simulink model "modules"  (R2017a)
settings: Solver=ode4  StartTime=0.0  StopTime=time_stop  FixedStep=time_step  RelTol=1e-3
values from neighbouring files (symbols this model uses):
  psi = state(3)    [PSVobstacleShip_class.m]    (also in PSVvessel_class.m = obj.eta(3); PsiReferenceModel_class.m = obj.desired_psi_vector; SBMPC_PSVvessel_class.m = obj.eta(3))
undefined symbols (not defined in the file or in its folder): beta, Delta_guidance, Delta_matrix, eta_initial, initial_desired_psi_vector, initial_desired_u_vector, initial_next_waypoint_indexes, initial_obstacle_ship_states, initial_obstacle_ship_states_dot, initial_reference_psi_vector, initial_reference_u_vector, initial_SBMPC_desired_psi_vector, initial_SBMPC_desired_u_vector, initial_SBMPC_next_waypoint_indexes, initial_SBMPC_obstacle_ship_states, initial_SBMPC_obstacle_ship_states_dot, initial_SBMPC_reference_psi_vector, initial_SBMPC_reference_u_vector, initial_SBMPC_x_d_psi_matrix, initial_SBMPC_x_d_u_matrix, initial_state, initial_x_d_psi_matrix, initial_x_d_u_matrix, K_sway, K_yaw, Kp_feedback_linearization, kp_heading, Nmax, nu_initial, num_obs_ship_waypoints, num_prediction_time_steps, number_of_control_behaviors, number_of_obstacle_ships, number_of_SBMPC_obstacle_ships, obs_speed_between_waypoints, obstacle_waypoint_matrix, Omega_matrix, own_ship_reference_psi_init, own_ship_reference_speed, Psi_init, radius_of_acceptance, SBMPC_obs_speed_between_waypoints, SBMPC_obstacle_waypoint_matrix, seconds_between_prediction, state_vector_init, T, T_k_surge, T_k_sway, T_k_yaw, T_s, T_waypoints, time_step, tsamp, U, U_init, V_init, waypoints_obstacle_ships, waypoints_own_ship, Xmax, Ymax
(part 2 of 5)

== system modules/obstacle ships/guidance  ==
  state matrix : Inport
  "waypoints matrix " : Inport  Port=2
  MATLAB Function1 : MATLAB Function  TreatAsAtomicUnit=on
  Scope : Scope
  Scope1 : Scope
  Scope2 : Scope
  obstacle waypoint guidance : MATLAB Function  TreatAsAtomicUnit=on
  "reference psi " : Outport
  reference u vector : Outport  Port=2
  "next_waypoints_indexes " : Outport  Port=3
  wires:
  "waypoints matrix "/1 -> obstacle waypoint guidance/1(obstacle_waypoints)
  state matrix/1 -> obstacle waypoint guidance/2(state_matrix)
  obstacle waypoint guidance/1(reference_psi_vector) -> "reference psi "/1, Scope/1
  MATLAB Function1/1(u_vector) -> Scope2/1, reference u vector/1
  obstacle waypoint guidance/2(next_waypoints_indexes) -> MATLAB Function1/1(next_waypoints_indexes), Scope1/1, "next_waypoints_indexes "/1

== system modules/obstacle ships/reference model for psi ==
  note: row vector
  note: row vector
  reference psi vector : Inport
  Scope3 : Scope  NumInputPorts=2
  To Workspace : ToWorkspace  VariableName=obstacle_ships_reference_psi_vector  SampleTime=tsamp
      settings: Save2DSignal=2-D array (concatenate along first dimension)
  To Workspace1 : ToWorkspace  VariableName=obstacle_ships_desired_psi_vector  SampleTime=tsamp
      settings: Save2DSignal=2-D array (concatenate along first dimension)
  "psi reference model " : MATLAB Function  TreatAsAtomicUnit=on
  "desired psi vector " : Outport
  wires:
  "psi reference model "/1(desired_psi_vector) -> Scope3/1, To Workspace1/1, "desired psi vector "/1
  reference psi vector/1 -> Scope3/2, To Workspace/1, "psi reference model "/1(reference_psi_vector)

== system modules/obstacle ships/reference model for u ==
  note: row vector
  note: row vector
  "reference u vector " : Inport
  MATLAB Function1 : MATLAB Function  TreatAsAtomicUnit=on
  To Workspace : ToWorkspace  VariableName=obstacle_ships_reference_u_vector  SampleTime=tsamp
      settings: Save2DSignal=2-D array (concatenate along first dimension)
  To Workspace1 : ToWorkspace  VariableName=obstacle_ships_desired_u_vector  SampleTime=tsamp
      settings: Save2DSignal=2-D array (concatenate along first dimension)
  desired_u_vector : Outport
  wires:
  "reference u vector "/1 -> To Workspace/1, MATLAB Function1/1(reference_u_vetor)
  MATLAB Function1/1(desired_u_vector) -> To Workspace1/1, desired_u_vector/1

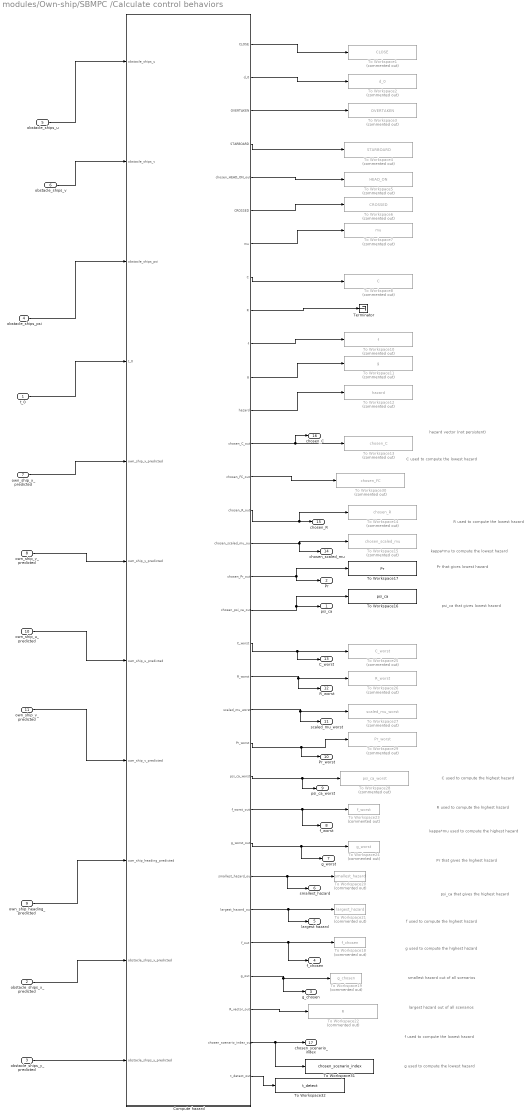
== system modules/Own-ship/SBMPC /Calculate control behaviors ==
  note: hazard vector (not persistent)
  note: C used to compute the lowest hazard
  note: R used to compute the lowest hazard
  note: kappa*mu to compute the lowest hazard
  note: Pr that gives lowest hazard
  note: psi_ca that gives lowest hazard
  note: C used to compute the highest hazard
  note: R used to compute the highest hazard
  note: kappa*mu used to compute the highest hazard
  note: Pr that gives the highest hazard
  note: psi_ca that gives the highest hazard
  note: f used to compute the highest hazard
  note: g used to compute the highest hazard
  note: smallest hazard out of all scenarios
  note: largest hazard out of all scenarios
  note: f used to compute the lowest hazard
  note: g used to compute the lowest hazard
  t_0 : Inport
  obstacle_ships_x_predicted : Inport  Port=2  SampleTime=time_step
      settings: VarSizeSig=Yes
  "obstacle_ships_y_predicted " : Inport  Port=3  SampleTime=time_step
      settings: VarSizeSig=Yes
  obstacle_ships_psi : Inport  Port=4
  obstacle_ships_u : Inport  Port=5
  obstacle_ships_v : Inport  Port=6
  own_ship_x_predicted : Inport  Port=7  SampleTime=time_step
      settings: VarSizeSig=Yes
  own_ship_y_predicted : Inport  Port=8  SampleTime=time_step
      settings: VarSizeSig=Yes
  "own_ship_heading_predicted " : Inport  Port=9  SampleTime=time_step
      settings: VarSizeSig=Yes
  own_ship_u_predicted : Inport  Port=10  SampleTime=time_step
      settings: VarSizeSig=Yes
  "own_ship_v_predicted " : Inport  Port=11  SampleTime=time_step
      settings: VarSizeSig=Yes
  Compute hazard : MATLAB Function  TreatAsAtomicUnit=on
  Terminator : Terminator
  To Workspace1 : ToWorkspace  Commented=on  VariableName=CLOSE  SaveFormat=Structure With Time  SampleTime=tsamp
  To Workspace10 : ToWorkspace  Commented=on  VariableName=f  SaveFormat=Structure With Time  SampleTime=tsamp
      settings: Save2DSignal=2-D array (concatenate along first dimension)
  To Workspace11 : ToWorkspace  Commented=on  VariableName=g  SaveFormat=Structure With Time  SampleTime=tsamp
  To Workspace12 : ToWorkspace  Commented=on  VariableName=hazard  SaveFormat=Structure With Time  SampleTime=tsamp
      settings: Save2DSignal=2-D array (concatenate along first dimension)
  To Workspace13 : ToWorkspace  Commented=on  VariableName=chosen_C  SampleTime=tsamp
      settings: Save2DSignal=2-D array (concatenate along first dimension)
  To Workspace14 : ToWorkspace  Commented=on  VariableName=chosen_R  SampleTime=tsamp
      settings: Save2DSignal=2-D array (concatenate along first dimension)
  To Workspace15 : ToWorkspace  Commented=on  VariableName=chosen_scaled_mu  SampleTime=tsamp
      settings: Save2DSignal=2-D array (concatenate along first dimension)
  To Workspace16 : ToWorkspace  VariableName=psi_ca  SampleTime=tsamp
      settings: Save2DSignal=2-D array (concatenate along first dimension)
  To Workspace17 : ToWorkspace  VariableName=Pr  SampleTime=tsamp
      settings: Save2DSignal=2-D array (concatenate along first dimension)
  To Workspace18 : ToWorkspace  Commented=on  VariableName=f_chosen  SampleTime=tsamp
      settings: Save2DSignal=2-D array (concatenate along first dimension)
  To Workspace19 : ToWorkspace  Commented=on  VariableName=g_chosen  SampleTime=tsamp
      settings: Save2DSignal=2-D array (concatenate along first dimension)
  To Workspace2 : ToWorkspace  Commented=on  VariableName=d_0  SaveFormat=Structure With Time  SampleTime=tsamp
  To Workspace20 : ToWorkspace  Commented=on  VariableName=smallest_hazard  SampleTime=tsamp
      settings: Save2DSignal=2-D array (concatenate along first dimension)
  To Workspace21 : ToWorkspace  Commented=on  VariableName=largest_hazard  SampleTime=tsamp
      settings: Save2DSignal=2-D array (concatenate along first dimension)
  To Workspace22 : ToWorkspace  Commented=on  VariableName=R  SaveFormat=Structure With Time  SampleTime=tsamp
  To Workspace23 : ToWorkspace  Commented=on  VariableName=f_worst  SampleTime=tsamp
      settings: Save2DSignal=2-D array (concatenate along first dimension)
  To Workspace24 : ToWorkspace  Commented=on  VariableName=g_worst  SampleTime=tsamp
      settings: Save2DSignal=2-D array (concatenate along first dimension)
  To Workspace25 : ToWorkspace  Commented=on  VariableName=C_worst  SampleTime=tsamp
      settings: Save2DSignal=2-D array (concatenate along first dimension)
  To Workspace26 : ToWorkspace  Commented=on  VariableName=R_worst  SampleTime=tsamp
      settings: Save2DSignal=2-D array (concatenate along first dimension)
  To Workspace27 : ToWorkspace  Commented=on  VariableName=scaled_mu_worst  SampleTime=tsamp
      settings: Save2DSignal=2-D array (concatenate along first dimension)
  To Workspace28 : ToWorkspace  Commented=on  VariableName=psi_ca_worst  SampleTime=tsamp
      settings: Save2DSignal=2-D array (concatenate along first dimension)
  To Workspace29 : ToWorkspace  Commented=on  VariableName=Pr_worst  SampleTime=tsamp
      settings: Save2DSignal=2-D array (concatenate along first dimension)
  To Workspace3 : ToWorkspace  Commented=on  VariableName=OVERTAKEN  SaveFormat=Structure With Time  SampleTime=tsamp
  To Workspace30 : ToWorkspace  Commented=on  VariableName=chosen_FC  SampleTime=tsamp
      settings: Save2DSignal=2-D array (concatenate along first dimension)
  To Workspace31 : ToWorkspace  VariableName=chosen_scenario_index  SampleTime=tsamp
      settings: Save2DSignal=2-D array (concatenate along first dimension)
  To Workspace32 : ToWorkspace  VariableName=t_detect  SaveFormat=Structure With Time  SampleTime=tsamp
      settings: Save2DSignal=2-D array (concatenate along first dimension)
  To Workspace4 : ToWorkspace  Commented=on  VariableName=STARBOARD  SaveFormat=Structure With Time  SampleTime=tsamp
  To Workspace5 : ToWorkspace  Commented=on  VariableName=HEAD_ON  SaveFormat=Structure With Time  SampleTime=tsamp
      settings: Save2DSignal=2-D array (concatenate along first dimension)
  To Workspace6 : ToWorkspace  Commented=on  VariableName=CROSSED  SaveFormat=Structure With Time  SampleTime=tsamp
  To Workspace7 : ToWorkspace  Commented=on  VariableName=mu  SaveFormat=Structure With Time  SampleTime=tsamp
  To Workspace8 : ToWorkspace  Commented=on  VariableName=C  SampleTime=tsamp
  psi_ca : Outport  SampleTime=time_step
  Pr : Outport  Port=2  SampleTime=time_step
  "g_chosen " : Outport  Port=3  SampleTime=time_step
  f_chosen : Outport  Port=4  SampleTime=time_step
  largest hazard : Outport  Port=5  SampleTime=time_step
  smallest_hazard : Outport  Port=6  SampleTime=time_step
  "g_worst " : Outport  Port=7  SampleTime=time_step
  f_worst : Outport  Port=8  SampleTime=time_step
  psi_ca_worst : Outport  Port=9  SampleTime=time_step
  Pr_worst : Outport  Port=10  SampleTime=time_step
  scaled_mu_worst : Outport  Port=11  SampleTime=time_step
  R_worst : Outport  Port=12  SampleTime=time_step
  C_worst : Outport  Port=13  SampleTime=time_step
  chosen_scaled_mu : Outport  Port=14  SampleTime=time_step
  chosen_R : Outport  Port=15  SampleTime=time_step
  chosen_C : Outport  Port=16  SampleTime=time_step
  "chosen_scenario_index " : Outport  Port=17  SampleTime=time_step
  wires:
  own_ship_x_predicted/1 -> Compute hazard/5(own_ship_x_predicted)
  own_ship_y_predicted/1 -> Compute hazard/6(own_ship_y_predicted)
  obstacle_ships_x_predicted/1 -> Compute hazard/10(obstacle_ships_x_predicted)
  "obstacle_ships_y_predicted "/1 -> Compute hazard/11(obstacle_ships_y_predicted)
  t_0/1 -> Compute hazard/4(t_0)
  Compute hazard/1(CLOSE) -> To Workspace1/1
  Compute hazard/2(d_0) -> To Workspace2/1
  obstacle_ships_v/1 -> Compute hazard/2(obstacle_ships_v)
  obstacle_ships_u/1 -> Compute hazard/1(obstacle_ships_u)
  own_ship_u_predicted/1 -> Compute hazard/7(own_ship_u_predicted)
  "own_ship_v_predicted "/1 -> Compute hazard/8(own_ship_v_predicted)
  "own_ship_heading_predicted "/1 -> Compute hazard/9(own_ship_heading_predicted)
  obstacle_ships_psi/1 -> Compute hazard/3(obstacle_ships_psi)
  Compute hazard/3(OVERTAKEN) -> To Workspace3/1
  Compute hazard/4(STARBOARD) -> To Workspace4/1
  Compute hazard/5(chosen_HEAD_ON_out) -> To Workspace5/1
  Compute hazard/6(CROSSED) -> To Workspace6/1
  Compute hazard/7(mu) -> To Workspace7/1
  Compute hazard/12(hazard) -> To Workspace12/1
  Compute hazard/8(C) -> To Workspace8/1
  Compute hazard/10(f) -> To Workspace10/1
  Compute hazard/11(g) -> To Workspace11/1
  Compute hazard/13(chosen_C_out) -> chosen_C/1, To Workspace13/1
  Compute hazard/15(chosen_R_out) -> To Workspace14/1, chosen_R/1
  Compute hazard/16(chosen_scaled_mu_out) -> To Workspace15/1, chosen_scaled_mu/1
  Compute hazard/18(chosen_psi_ca_out) -> To Workspace16/1, psi_ca/1
  Compute hazard/19(C_worst) -> C_worst/1, To Workspace25/1
  Compute hazard/20(R_worst) -> R_worst/1, To Workspace26/1
  Compute hazard/21(scaled_mu_worst) -> scaled_mu_worst/1, To Workspace27/1
  Compute hazard/22(Pr_worst) -> Pr_worst/1, To Workspace29/1
  Compute hazard/23(psi_ca_worst) -> psi_ca_worst/1, To Workspace28/1
  Compute hazard/25(g_worst_out) -> "g_worst "/1, To Workspace24/1
  Compute hazard/24(f_worst_out) -> f_worst/1, To Workspace23/1
  Compute hazard/17(chosen_Pr_out) -> To Workspace17/1, Pr/1
  Compute hazard/28(f_out) -> f_chosen/1, To Workspace18/1
  Compute hazard/29(g_out) -> "g_chosen "/1, To Workspace19/1
  Compute hazard/26(smallest_hazard_out) -> smallest_hazard/1, To Workspace20/1
  Compute hazard/27(largest_hazard_out) -> largest hazard/1, To Workspace21/1
  Compute hazard/30(R_vector_out) -> To Workspace22/1
  Compute hazard/9(R) -> Terminator/1
  Compute hazard/14(chosen_FC_out) -> To Workspace30/1
  Compute hazard/31(chosen_scenario_index_out) -> To Workspace31/1, "chosen_scenario_index "/1
  Compute hazard/32(t_detect_out) -> To Workspace32/1

== system modules/Own-ship/SBMPC /Own-ship trajectory prediction ==
  note: each row = time step in prediction horizion
      | each column = a different control scenario
  note: each row = time step in prediction horizion
      | each column = a different control scenario
  note: each row = time step in prediction horizion
      | each column = a different control scenario
  note: each row = time step in prediction horizion
      | each column = a different control scenario
  note: each row = time step in prediction horizion
      | each column = a different control scenario
  t_0 : Inport
  waypoints_matrix : Inport  Port=2
  "eta_initial " : Inport  Port=3
  nu_initial : Inport  Port=4
  next_waypoint_index : Inport  Port=5
  Own ship trajectory prediction : MATLAB Function  TreatAsAtomicUnit=on
  To Workspace1 : ToWorkspace  Commented=on  VariableName=own_ship_x_predicted  SaveFormat=Structure With Time  SampleTime=tsamp
  To Workspace3 : ToWorkspace  Commented=on  VariableName=own_ship_y_predicted  SaveFormat=Structure With Time  SampleTime=tsamp
  To Workspace4 : ToWorkspace  Commented=on  VariableName=own_ship_heading_predicted  SaveFormat=Structure With Time  SampleTime=tsamp
  To Workspace5 : ToWorkspace  Commented=on  VariableName=own_ship_u_predicted  SaveFormat=Structure With Time  SampleTime=tsamp
  To Workspace6 : ToWorkspace  Commented=on  VariableName=own_ship_v_predicted  SaveFormat=Structure With Time  SampleTime=tsamp
  own_ship_x_predicted : Outport  SampleTime=time_step
  own_ship_y_predicted : Outport  Port=2  SampleTime=time_step
  own_ship_heading_predicted : Outport  Port=3  SampleTime=time_step
  own_ship_u_predicted : Outport  Port=4  SampleTime=time_step
  "own_ship_v_predicted " : Outport  Port=5  SampleTime=time_step
  wires:
  waypoints_matrix/1 -> Own ship trajectory prediction/4(waypoints_matrix)
  nu_initial/1 -> Own ship trajectory prediction/3(nu_initial)
  "eta_initial "/1 -> Own ship trajectory prediction/2(eta_initial)
  next_waypoint_index/1 -> Own ship trajectory prediction/5(next_waypoint_index)
  t_0/1 -> Own ship trajectory prediction/1(t_0)
  Own ship trajectory prediction/1(own_ship_x_predicted) -> own_ship_x_predicted/1, To Workspace1/1
  Own ship trajectory prediction/2(own_ship_y_predicted) -> own_ship_y_predicted/1, To Workspace3/1
  Own ship trajectory prediction/3(own_ship_heading_predicted) -> To Workspace4/1, own_ship_heading_predicted/1
  Own ship trajectory prediction/4(own_ship_u_predicted) -> own_ship_u_predicted/1, To Workspace5/1
  Own ship trajectory prediction/5(own_ship_v_predicted) -> "own_ship_v_predicted "/1, To Workspace6/1

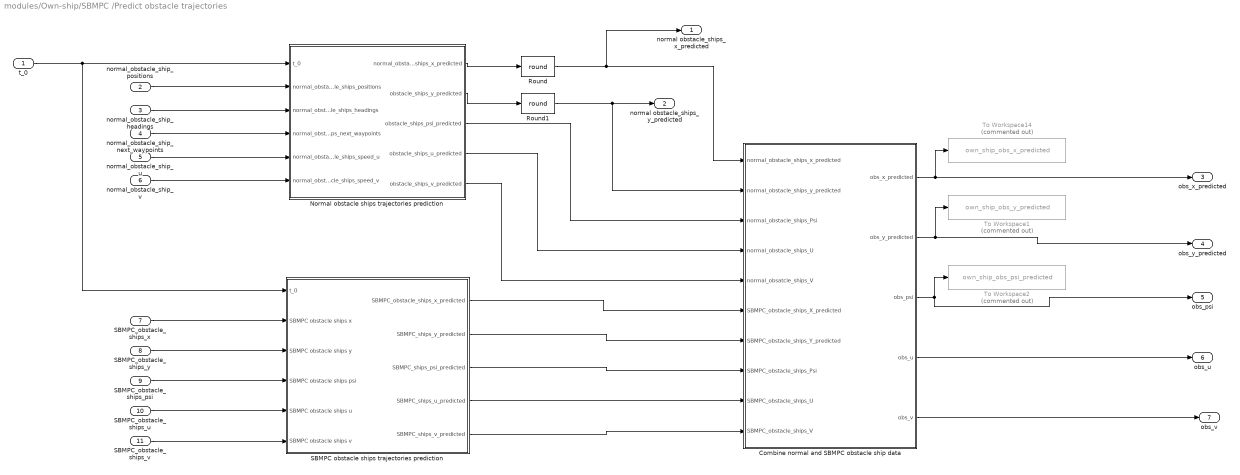
== system modules/Own-ship/SBMPC /Predict obstacle trajectories ==
  t_0 : Inport
  normal_obstacle_ship_positions : Inport  Port=2
  normal_obstacle_ship_headings : Inport  Port=3
  normal_obstacle_ship_next_waypoints : Inport  Port=4
  normal_obstacle_ship_u : Inport  Port=5
  normal_obstacle_ship_v : Inport  Port=6
  SBMPC_obstacle_ships_x : Inport  Port=7
  SBMPC_obstacle_ships_y : Inport  Port=8
  SBMPC_obstacle_ships_psi : Inport  Port=9
  SBMPC_obstacle_ships_u : Inport  Port=10
  SBMPC_obstacle_ships_v : Inport  Port=11
  "Combine normal and SBMPC obstacle ship data " : MATLAB Function  TreatAsAtomicUnit=on
  Normal obstacle ships trajectories prediction : Subsystem
  Round : Rounding  Operator=round
  Round1 : Rounding  Operator=round
  SBMPC obstacle ships trajectories prediction : Subsystem
  To Workspace1 : ToWorkspace  Commented=on  VariableName=own_ship_obs_y_predicted  SaveFormat=Structure With Time  SampleTime=tsamp
      settings: Save2DSignal=2-D array (concatenate along first dimension)
  To Workspace14 : ToWorkspace  Commented=on  VariableName=own_ship_obs_x_predicted  SaveFormat=Structure With Time  SampleTime=tsamp
      settings: Save2DSignal=2-D array (concatenate along first dimension)
  To Workspace2 : ToWorkspace  Commented=on  VariableName=own_ship_obs_psi_predicted  SaveFormat=Structure With Time  SampleTime=tsamp
      settings: Save2DSignal=2-D array (concatenate along first dimension)
  normal obstacle_ships_x_predicted : Outport  SampleTime=time_step
  "normal obstacle_ships_y_predicted " : Outport  Port=2  SampleTime=time_step
  obs_x_predicted : Outport  Port=3
  obs_y_predicted : Outport  Port=4
  obs_psi : Outport  Port=5
  obs_u : Outport  Port=6
  obs_v : Outport  Port=7
  wires:
  Normal obstacle ships trajectories prediction/1(normal_obstacle_ships_x_predicted) -> Round/1
  normal_obstacle_ship_u/1 -> Normal obstacle ships trajectories prediction/5(normal_obstacle_ships_speed_u)
  normal_obstacle_ship_headings/1 -> Normal obstacle ships trajectories prediction/3(normal_obstacle_ships_headings)
  normal_obstacle_ship_positions/1 -> Normal obstacle ships trajectories prediction/2(normal_obstacle_ships_positions)
  Normal obstacle ships trajectories prediction/2(obstacle_ships_y_predicted) -> Round1/1
  normal_obstacle_ship_v/1 -> Normal obstacle ships trajectories prediction/6(normal_obstacle_ships_speed_v)
  "Combine normal and SBMPC obstacle ship data "/5(obs_v) -> obs_v/1
  Normal obstacle ships trajectories prediction/5(obstacle_ships_v_predicted) -> "Combine normal and SBMPC obstacle ship data "/5(normal_obsatcle_ships_V)
  Normal obstacle ships trajectories prediction/4(obstacle_ships_u_predicted) -> "Combine normal and SBMPC obstacle ship data "/4(normal_obstacle_ships_U)
  "Combine normal and SBMPC obstacle ship data "/2(obs_y_predicted) -> obs_y_predicted/1, To Workspace1/1
  "Combine normal and SBMPC obstacle ship data "/1(obs_x_predicted) -> obs_x_predicted/1, To Workspace14/1
  "Combine normal and SBMPC obstacle ship data "/3(obs_psi) -> obs_psi/1, To Workspace2/1
  normal_obstacle_ship_next_waypoints/1 -> Normal obstacle ships trajectories prediction/4(normal_obstacle_ships_next_waypoints)
  Normal obstacle ships trajectories prediction/3(obstacle_ships_psi_predicted) -> "Combine normal and SBMPC obstacle ship data "/3(normal_obstacle_ships_Psi)
  "Combine normal and SBMPC obstacle ship data "/4(obs_u) -> obs_u/1
  SBMPC_obstacle_ships_psi/1 -> SBMPC obstacle ships trajectories prediction/4(SBMPC obstacle ships psi)
  SBMPC_obstacle_ships_u/1 -> SBMPC obstacle ships trajectories prediction/5(SBMPC obstacle ships u)
  SBMPC_obstacle_ships_y/1 -> SBMPC obstacle ships trajectories prediction/3("SBMPC obstacle ships y ")
  SBMPC_obstacle_ships_v/1 -> SBMPC obstacle ships trajectories prediction/6(SBMPC obstacle ships v)
  SBMPC obstacle ships trajectories prediction/3(SBMPC_ships_psi_predicted) -> "Combine normal and SBMPC obstacle ship data "/8(SBMPC_obstacle_ships_Psi)
  SBMPC obstacle ships trajectories prediction/5(SBMPC_ships_v_predicted) -> "Combine normal and SBMPC obstacle ship data "/10(SBMPC_obstacle_ships_V)
  SBMPC obstacle ships trajectories prediction/4(SBMPC_ships_u_predicted) -> "Combine normal and SBMPC obstacle ship data "/9(SBMPC_obstacle_ships_U)
  SBMPC obstacle ships trajectories prediction/2(SBMPC_ships_y_predicted) -> "Combine normal and SBMPC obstacle ship data "/7(SBMPC_obstacle_ships_Y_predicted)
  SBMPC obstacle ships trajectories prediction/1(SBMPC_obstacle_ships_x_predicted) -> "Combine normal and SBMPC obstacle ship data "/6(SBMPC_obstacle_ships_X_predicted)
  SBMPC_obstacle_ships_x/1 -> SBMPC obstacle ships trajectories prediction/2("SBMPC obstacle ships x ")
  t_0/1 -> SBMPC obstacle ships trajectories prediction/1(t_0), Normal obstacle ships trajectories prediction/1(t_0)
  Round/1 -> normal obstacle_ships_x_predicted/1, "Combine normal and SBMPC obstacle ship data "/1(normal_obstacle_ships_x_predicted)
  Round1/1 -> "normal obstacle_ships_y_predicted "/1, "Combine normal and SBMPC obstacle ship data "/2(normal_obstacle_ships_y_predicted)

== system modules/Own-ship/vessel1/Vessel model ==
  desired_nu : Inport
  desired_psi : Inport  Port=2
  Pr : Inport  Port=3
  psi_ca : Inport  Port=4
  Demux : Demux  Outputs=6
  MATLAB Function : MATLAB Function  TreatAsAtomicUnit=on
  Mux : Mux  Inputs=3
  Terminator : Terminator
  To Workspace : ToWorkspace  Commented=on  VariableName=tau  SampleTime=tsamp
      settings: Save2DSignal=2-D array (concatenate along first dimension)
  state : Outport
  x : Outport  Port=2
  y : Outport  Port=3
  psi : Outport  Port=4
  u : Outport  Port=5
  v : Outport  Port=6
  r : Outport  Port=7
  wires:
  Demux/4 -> u/1, Mux/1
  Mux/1 -> Terminator/1  "nu"
  MATLAB Function/1(state) -> Demux/1, state/1
  Demux/5 -> v/1, Mux/2
  Demux/2 -> y/1
  Demux/6 -> r/1, Mux/3
  Demux/1 -> x/1
  Demux/3 -> psi/1
  desired_psi/1 -> MATLAB Function/4(desired_psi)
  desired_nu/1 -> MATLAB Function/3(desired_nu)
  MATLAB Function/2(tau) -> To Workspace/1
  psi_ca/1 -> MATLAB Function/2(psi_ca)
  Pr/1 -> MATLAB Function/1(Pr)

== system modules/Own-ship/vessel1/derivative ==
  desired_nu : Inport
  Memory2 : Memory
  vector derivative : MATLAB Function  TreatAsAtomicUnit=on
  desired_nu_dot : Outport
  wires:
  Memory2/1 -> vector derivative/2(x_previous)
  desired_nu/1 -> Memory2/1, vector derivative/1(x)
  vector derivative/1(derivative) -> desired_nu_dot/1

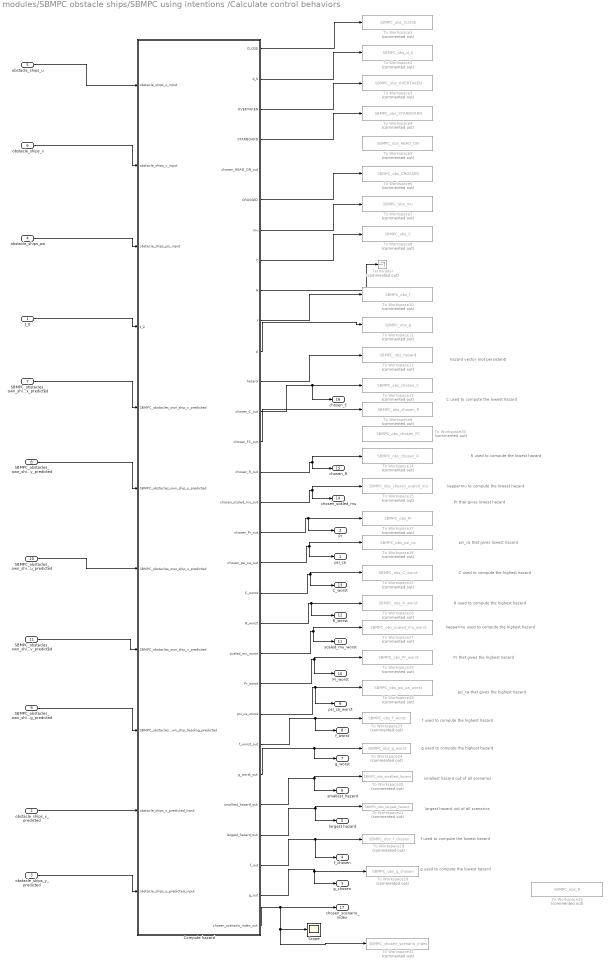
== system modules/SBMPC obstacle ships/SBMPC using intentions /Calculate control behaviors ==
  note: hazard vector (not persistent)
  note: C used to compute the lowest hazard
  note: R used to compute the lowest hazard
  note: kappa*mu to compute the lowest hazard
  note: Pr that gives lowest hazard
  note: psi_ca that gives lowest hazard
  note: C used to compute the highest hazard
  note: R used to compute the highest hazard
  note: kappa*mu used to compute the highest hazard
  note: Pr that gives the highest hazard
  note: psi_ca that gives the highest hazard
  note: f used to compute the highest hazard
  note: g used to compute the highest hazard
  note: smallest hazard out of all scenarios
  note: largest hazard out of all scenarios
  note: f used to compute the lowest hazard
  note: g used to compute the lowest hazard
  t_0 : Inport
  obstacle_ships_x_predicted : Inport  Port=2  SampleTime=time_step
      settings: VarSizeSig=Yes
  "obstacle_ships_y_predicted " : Inport  Port=3  SampleTime=time_step
      settings: VarSizeSig=Yes
  obstacle_ships_psi : Inport  Port=4
  obstacle_ships_u : Inport  Port=5
  obstacle_ships_v : Inport  Port=6
  SBMPC_obstacles_own_ship_x_predicted : Inport  Port=7  SampleTime=time_step
      settings: VarSizeSig=Yes
  SBMPC_obstacles_own_ship_y_predicted : Inport  Port=8  SampleTime=time_step
      settings: VarSizeSig=Yes
  "SBMPC_obstacles_own_ship_heading_predicted " : Inport  Port=9  SampleTime=time_step
      settings: VarSizeSig=Yes
  SBMPC_obstacles_own_ship_u_predicted : Inport  Port=10  SampleTime=time_step
      settings: VarSizeSig=Yes
  "SBMPC_obstacles_own_ship_v_predicted " : Inport  Port=11  SampleTime=time_step
      settings: VarSizeSig=Yes
  Compute hazard : MATLAB Function  TreatAsAtomicUnit=on
  Scope : Scope
  Terminator : Terminator  Commented=on
  To Workspace1 : ToWorkspace  Commented=on  VariableName=SBMPC_obs_CLOSE  SampleTime=tsamp
  To Workspace10 : ToWorkspace  Commented=on  VariableName=SBMPC_obs_f  SampleTime=tsamp
      settings: Save2DSignal=2-D array (concatenate along first dimension)
  To Workspace11 : ToWorkspace  Commented=on  VariableName=SBMPC_obs_g  SampleTime=tsamp
  To Workspace12 : ToWorkspace  Commented=on  VariableName=SBMPC_obs_hazard  SaveFormat=Structure With Time  SampleTime=tsamp
      settings: Save2DSignal=2-D array (concatenate along first dimension)
  To Workspace13 : ToWorkspace  Commented=on  VariableName=SBMPC_obs_chosen_C  SaveFormat=Structure With Time  SampleTime=tsamp
      settings: Save2DSignal=2-D array (concatenate along first dimension)
  To Workspace14 : ToWorkspace  Commented=on  VariableName=SBMPC_obs_chosen_R  SaveFormat=Structure With Time  SampleTime=tsamp
      settings: Save2DSignal=2-D array (concatenate along first dimension)
  To Workspace15 : ToWorkspace  Commented=on  VariableName=SBMPC_obs_chosen_scaled_mu  SaveFormat=Structure With Time  SampleTime=tsamp
      settings: Save2DSignal=2-D array (concatenate along first dimension)
  To Workspace16 : ToWorkspace  Commented=on  VariableName=SBMPC_obs_psi_ca  SaveFormat=Structure With Time  SampleTime=tsamp
      settings: Save2DSignal=2-D array (concatenate along first dimension)
  To Workspace17 : ToWorkspace  Commented=on  VariableName=SBMPC_obs_Pr  SaveFormat=Structure With Time  SampleTime=tsamp
      settings: Save2DSignal=2-D array (concatenate along first dimension)
  To Workspace18 : ToWorkspace  Commented=on  VariableName=SBMPC_obs_f_chosen  SaveFormat=Structure With Time  SampleTime=tsamp
      settings: Save2DSignal=2-D array (concatenate along first dimension)
  To Workspace19 : ToWorkspace  Commented=on  VariableName=SBMPC_obs_g_chosen  SaveFormat=Structure With Time  SampleTime=tsamp
      settings: Save2DSignal=2-D array (concatenate along first dimension)
  To Workspace2 : ToWorkspace  Commented=on  VariableName=SBMPC_obs_d_0  SampleTime=tsamp
  To Workspace20 : ToWorkspace  Commented=on  VariableName=SBMPC_obs_smallest_hazard  SaveFormat=Structure With Time  SampleTime=tsamp
      settings: Save2DSignal=2-D array (concatenate along first dimension)
  To Workspace21 : ToWorkspace  Commented=on  VariableName=SBMPC_obs_largest_hazard  SaveFormat=Structure With Time  SampleTime=tsamp
      settings: Save2DSignal=2-D array (concatenate along first dimension)
  To Workspace22 : ToWorkspace  Commented=on  VariableName=SBMPC_obs_R  SaveFormat=Structure With Time  SampleTime=tsamp
  To Workspace23 : ToWorkspace  Commented=on  VariableName=SBMPC_obs_f_worst  SaveFormat=Structure With Time  SampleTime=tsamp
      settings: Save2DSignal=2-D array (concatenate along first dimension)
  To Workspace24 : ToWorkspace  Commented=on  VariableName=SBMPC_obs_g_worst  SaveFormat=Structure With Time  SampleTime=tsamp
      settings: Save2DSignal=2-D array (concatenate along first dimension)
  To Workspace25 : ToWorkspace  Commented=on  VariableName=SBMPC_obs_C_worst  SaveFormat=Structure With Time  SampleTime=tsamp
      settings: Save2DSignal=2-D array (concatenate along first dimension)
  To Workspace26 : ToWorkspace  Commented=on  VariableName=SBMPC_obs_R_worst  SaveFormat=Structure With Time  SampleTime=tsamp
      settings: Save2DSignal=2-D array (concatenate along first dimension)
  To Workspace27 : ToWorkspace  Commented=on  VariableName=SBMPC_obs_scaled_mu_worst  SaveFormat=Structure With Time  SampleTime=tsamp
      settings: Save2DSignal=2-D array (concatenate along first dimension)
  To Workspace28 : ToWorkspace  Commented=on  VariableName=SBMPC_obs_psi_ca_worst  SaveFormat=Structure With Time  SampleTime=tsamp
      settings: Save2DSignal=2-D array (concatenate along first dimension)
  To Workspace29 : ToWorkspace  Commented=on  VariableName=SBMPC_obs_Pr_worst  SaveFormat=Structure With Time  SampleTime=tsamp
      settings: Save2DSignal=2-D array (concatenate along first dimension)
  To Workspace3 : ToWorkspace  Commented=on  VariableName=SBMPC_obs_OVERTAKEN  SampleTime=tsamp
  To Workspace30 : ToWorkspace  Commented=on  VariableName=SBMPC_obs_chosen_FC  SaveFormat=Structure With Time  SampleTime=tsamp
      settings: Save2DSignal=2-D array (concatenate along first dimension)
  To Workspace31 : ToWorkspace  Commented=on  VariableName=SBMPC_chosen_scenario_index  SaveFormat=Structure With Time  SampleTime=tsamp
      settings: Save2DSignal=2-D array (concatenate along first dimension)
  To Workspace4 : ToWorkspace  Commented=on  VariableName=SBMPC_obs_STARBOARD  SampleTime=tsamp
  To Workspace5 : ToWorkspace  Commented=on  VariableName=SBMPC_obs_HEAD_ON  SaveFormat=Structure With Time  SampleTime=tsamp
      settings: Save2DSignal=2-D array (concatenate along first dimension)
  To Workspace6 : ToWorkspace  Commented=on  VariableName=SBMPC_obs_CROSSED  SampleTime=tsamp
  To Workspace7 : ToWorkspace  Commented=on  VariableName=SBMPC_obs_mu  SampleTime=tsamp
  To Workspace8 : ToWorkspace  Commented=on  VariableName=SBMPC_obs_C  SampleTime=tsamp
  To Workspace9 : ToWorkspace  Commented=on  VariableName=SBMPC_obs_chosen_P  SaveFormat=Structure With Time  SampleTime=tsamp
      settings: Save2DSignal=2-D array (concatenate along first dimension)
  psi_ca : Outport  SampleTime=time_step
  Pr : Outport  Port=2  SampleTime=time_step
  "g_chosen " : Outport  Port=3  SampleTime=time_step
  f_chosen : Outport  Port=4  SampleTime=time_step
  largest hazard : Outport  Port=5  SampleTime=time_step
  smallest_hazard : Outport  Port=6  SampleTime=time_step
  "g_worst " : Outport  Port=7  SampleTime=time_step
  f_worst : Outport  Port=8  SampleTime=time_step
  psi_ca_worst : Outport  Port=9  SampleTime=time_step
  Pr_worst : Outport  Port=10  SampleTime=time_step
  scaled_mu_worst : Outport  Port=11  SampleTime=time_step
  R_worst : Outport  Port=12  SampleTime=time_step
  C_worst : Outport  Port=13  SampleTime=time_step
  chosen_scaled_mu : Outport  Port=14  SampleTime=time_step
  chosen_R : Outport  Port=15  SampleTime=time_step
  chosen_C : Outport  Port=16  SampleTime=time_step
  chosen_scenario_index : Outport  Port=17  SampleTime=time_step
  wires:
  SBMPC_obstacles_own_ship_x_predicted/1 -> Compute hazard/5(SBMPC_obstacles_own_ship_x_predicted)
  SBMPC_obstacles_own_ship_y_predicted/1 -> Compute hazard/6(SBMPC_obstacles_own_ship_y_predicted)
  obstacle_ships_x_predicted/1 -> Compute hazard/10(obstacle_ships_x_predicted_input)
  "obstacle_ships_y_predicted "/1 -> Compute hazard/11(obstacle_ships_y_predicted_input)
  t_0/1 -> Compute hazard/4(t_0)
  Compute hazard/1(CLOSE) -> To Workspace1/1
  Compute hazard/2(d_0) -> To Workspace2/1
  obstacle_ships_v/1 -> Compute hazard/2(obstacle_ships_v_input)
  obstacle_ships_u/1 -> Compute hazard/1(obstacle_ships_u_input)
  SBMPC_obstacles_own_ship_u_predicted/1 -> Compute hazard/7(SBMPC_obstacles_own_ship_u_predicted)
  "SBMPC_obstacles_own_ship_v_predicted "/1 -> Compute hazard/8(SBMPC_obstacles_own_ship_v_predicted)
  "SBMPC_obstacles_own_ship_heading_predicted "/1 -> Compute hazard/9(SBMPC_obstacles_own_ship_heading_predicted)
  obstacle_ships_psi/1 -> Compute hazard/3(obstacle_ships_psi_input)
  Compute hazard/3(OVERTAKEN) -> To Workspace3/1
  Compute hazard/4(STARBOARD) -> To Workspace4/1
  ? -> To Workspace5/1
  Compute hazard/6(CROSSED) -> To Workspace6/1
  Compute hazard/7(mu) -> To Workspace7/1
  Compute hazard/12(hazard) -> To Workspace12/1
  Compute hazard/8(C) -> To Workspace8/1
  Compute hazard/10(f) -> To Workspace10/1
  Compute hazard/11(g) -> To Workspace11/1
  Compute hazard/13(chosen_C_out) -> chosen_C/1, To Workspace13/1
  Compute hazard/15(chosen_R_out) -> To Workspace14/1, chosen_R/1
  Compute hazard/16(chosen_scaled_mu_out) -> To Workspace15/1, chosen_scaled_mu/1
  Compute hazard/18(chosen_psi_ca_out) -> To Workspace16/1, psi_ca/1
  Compute hazard/19(C_worst) -> To Workspace25/1, C_worst/1
  Compute hazard/20(R_worst) -> R_worst/1, To Workspace26/1
  Compute hazard/21(scaled_mu_worst) -> To Workspace27/1, scaled_mu_worst/1
  Compute hazard/22(Pr_worst) -> To Workspace29/1, Pr_worst/1
  Compute hazard/23(psi_ca_worst) -> psi_ca_worst/1, To Workspace28/1
  Compute hazard/25(g_worst_out) -> "g_worst "/1, To Workspace24/1
  Compute hazard/24(f_worst_out) -> f_worst/1, To Workspace23/1
  Compute hazard/17(chosen_Pr_out) -> To Workspace17/1, Pr/1
  Compute hazard/28(f_out) -> f_chosen/1, To Workspace18/1
  Compute hazard/29(g_out) -> "g_chosen "/1, To Workspace19/1
  Compute hazard/26(smallest_hazard_out) -> smallest_hazard/1, To Workspace20/1
  Compute hazard/27(largest_hazard_out) -> largest hazard/1, To Workspace21/1
  Compute hazard/9(R) -> Terminator/1
  Compute hazard/14(chosen_FC_out) -> To Workspace9/1
  ? -> To Workspace30/1
  Compute hazard/30(chosen_scenario_index_out) -> To Workspace31/1, Scope/1, chosen_scenario_index/1

== system modules/SBMPC obstacle ships/SBMPC using intentions /Normal obstacle ships trajectories prediction ==
  note: column vector, row = time step in prediction horizion and column = obstacle
  note: column vector, row = time step in prediction horizion and column = obstacle
  t_0 : Inport
  normal_obstacle_ships_positions : Inport  Port=2
  normal_obstacle_ships_headings : Inport  Port=3
  normal_obstacle_ships_next_waypoints : Inport  Port=4
  normal_obstacle_ships_u : Inport  Port=5
  normal_obstacle_ships_v : Inport  Port=6
  Normal obstacle ships trajectories prediction : MATLAB Function  TreatAsAtomicUnit=on
  Scope1 : Scope
  To Workspace1 : ToWorkspace  Commented=on  VariableName=normal_obstacle_ships_u_predicted  SaveFormat=Structure With Time  SampleTime=tsamp
  To Workspace2 : ToWorkspace  Commented=on  VariableName=normal_obstacle_ships_psi_predicted  SaveFormat=Structure With Time  SampleTime=tsamp
  To Workspace3 : ToWorkspace  Commented=on  VariableName=normal_obstacle_ships_y_predicted  SaveFormat=Structure With Time  SampleTime=tsamp
  To Workspace4 : ToWorkspace  Commented=on  VariableName=normal_obstacle_ships_x_predicted  SaveFormat=Structure With Time  SampleTime=tsamp
  To Workspace5 : ToWorkspace  Commented=on  VariableName=normal_obstacle_ships_v_predicted  SaveFormat=Structure With Time  SampleTime=tsamp
  normal_obstacle_ships_x_predicted : Outport  SampleTime=time_step
  obstacle_ships_y_predicted : Outport  Port=2  SampleTime=time_step
  obstacle_ships_psi_predicted : Outport  Port=3  SampleTime=time_step
  obstacle_ships_u_predicted : Outport  Port=4  SampleTime=time_step
  obstacle_ships_v_predicted : Outport  Port=5  SampleTime=time_step
  wires:
  normal_obstacle_ships_positions/1 -> Normal obstacle ships trajectories prediction/5(obstacle_ships_positions)
  t_0/1 -> Normal obstacle ships trajectories prediction/6(t_0)
  Normal obstacle ships trajectories prediction/1(obstacle_ships_x_predicted) -> normal_obstacle_ships_x_predicted/1, To Workspace4/1
  Normal obstacle ships trajectories prediction/2(obstacle_ships_y_predicted) -> obstacle_ships_y_predicted/1, To Workspace3/1
  normal_obstacle_ships_headings/1 -> Normal obstacle ships trajectories prediction/1(obstacle_ships_psi)
  normal_obstacle_ships_next_waypoints/1 -> Normal obstacle ships trajectories prediction/4(obstacle_ships_next_waypoint_index_vector), Scope1/1
  Normal obstacle ships trajectories prediction/5(obstacle_ships_psi_predicted) -> To Workspace2/1, obstacle_ships_psi_predicted/1
  Normal obstacle ships trajectories prediction/3(obstacle_ships_u_predicted) -> To Workspace1/1, obstacle_ships_u_predicted/1
  Normal obstacle ships trajectories prediction/4(obstacle_ships_v_predicted) -> To Workspace5/1, obstacle_ships_v_predicted/1
  normal_obstacle_ships_u/1 -> Normal obstacle ships trajectories prediction/2(obstacle_ships_u)
  normal_obstacle_ships_v/1 -> Normal obstacle ships trajectories prediction/3(obstacle_ships_v)

== system modules/SBMPC obstacle ships/SBMPC using intentions /SBMPC obstacles: own-ship trajectory prediction ==
  note: each row = time step in prediction horizion
      | each column = a different control scenario
  note: each row = time step in prediction horizion
      | each column = a different control scenario
  note: each row = time step in prediction horizion
      | each column = a different control scenario
  note: each row = time step in prediction horizion
      | each column = a different control scenario
  note: each row = time step in prediction horizion
      | each column = a different control scenario
  t_0 : Inport
  SBMPC_obs_waypoints_matrix : Inport  Port=2
  "SBMPC_obs_eta_initial " : Inport  Port=3
  SBMPC_obs_nu_initial : Inport  Port=4
  SBMPC_obs_next_waypoint_index : Inport  Port=5
  Own ship trajectory prediction : MATLAB Function  TreatAsAtomicUnit=on
  To Workspace1 : ToWorkspace  Commented=on  VariableName=SBMPC_own_ship_x_predicted  SaveFormat=Structure With Time  SampleTime=tsamp
  To Workspace3 : ToWorkspace  Commented=on  VariableName=SBMPC_own_ship_y_predicted  SaveFormat=Structure With Time  SampleTime=tsamp
  To Workspace4 : ToWorkspace  Commented=on  VariableName=SBMPC_own_ship_heading_predicted  SaveFormat=Structure With Time  SampleTime=tsamp
  To Workspace5 : ToWorkspace  Commented=on  VariableName=SBMPC_own_ship_u_predicted  SaveFormat=Structure With Time  SampleTime=tsamp
  To Workspace6 : ToWorkspace  Commented=on  VariableName=SBMPC_own_ship_v_predicted  SaveFormat=Structure With Time  SampleTime=tsamp
  SBMPC_obs_own_ship_x_predicted : Outport  SampleTime=time_step
  SBMPC_obs_own_ship_y_predicted : Outport  Port=2  SampleTime=time_step
  SBMPC_obs_own_ship_heading_predicted : Outport  Port=3  SampleTime=time_step
  SBMPC_obs_own_ship_u_predicted : Outport  Port=4  SampleTime=time_step
  "SBMPC_obs_own_ship_v_predicted " : Outport  Port=5  SampleTime=time_step
  wires:
  SBMPC_obs_waypoints_matrix/1 -> Own ship trajectory prediction/4(waypoints_matrix)
  SBMPC_obs_nu_initial/1 -> Own ship trajectory prediction/3(nu_initial)
  "SBMPC_obs_eta_initial "/1 -> Own ship trajectory prediction/2(eta_initial)
  SBMPC_obs_next_waypoint_index/1 -> Own ship trajectory prediction/5(next_waypoint_index)
  t_0/1 -> Own ship trajectory prediction/1(t_0)
  Own ship trajectory prediction/1(own_ship_x_predicted) -> SBMPC_obs_own_ship_x_predicted/1, To Workspace1/1
  Own ship trajectory prediction/2(own_ship_y_predicted) -> SBMPC_obs_own_ship_y_predicted/1, To Workspace3/1
  Own ship trajectory prediction/3(own_ship_heading_predicted) -> To Workspace4/1, SBMPC_obs_own_ship_heading_predicted/1
  Own ship trajectory prediction/4(own_ship_u_predicted) -> SBMPC_obs_own_ship_u_predicted/1, To Workspace5/1
  Own ship trajectory prediction/5(own_ship_v_predicted) -> "SBMPC_obs_own_ship_v_predicted "/1, To Workspace6/1

== system modules/SBMPC obstacle ships/SBMPC using intentions /own-ship obstacle ships trajectories prediction ==
  note: column vector, row = time step in prediction horizion and column = obstacle
  note: column vector, row = time step in prediction horizion and column = obstacle
  t_0 : Inport
  own_ship_obstacle_x : Inport  Port=2
  own_ship_obstacle_headings : Inport  Port=3
  own_ship_obstacle_u : Inport  Port=4
  own_ship_obstacle_v : Inport  Port=5
  own_ship_obstacle_y : Inport  Port=6
  Normal obstacle ships trajectories prediction : MATLAB Function  TreatAsAtomicUnit=on
  To Workspace1 : ToWorkspace  Commented=on  VariableName=own_ship_obstacle_ships_u_predicted  SaveFormat=Structure With Time  SampleTime=tsamp
  To Workspace2 : ToWorkspace  Commented=on  VariableName=own_ship_obstacle_ships_psi_predicted  SaveFormat=Structure With Time  SampleTime=tsamp
  To Workspace3 : ToWorkspace  Commented=on  VariableName=own_ship_obstacle_ships_y_predicted  SaveFormat=Structure With Time  SampleTime=tsamp
  To Workspace4 : ToWorkspace  Commented=on  VariableName=own_ship_obstacle_ships_x_predicted  SaveFormat=Structure With Time  SampleTime=tsamp
  To Workspace5 : ToWorkspace  Commented=on  VariableName=own_ship__obstacle_ships_v_predicted  SaveFormat=Structure With Time  SampleTime=tsamp
  own_ship_obstacle_x_predicted : Outport  SampleTime=time_step
  own_ship_obstacle_y_predicted : Outport  Port=2  SampleTime=time_step
  own_ship_obstacle_psi_predicted : Outport  Port=3  SampleTime=time_step
  own_ship_obstacle_u_predicted : Outport  Port=4  SampleTime=time_step
  own_ship_obstacle_v_predicted : Outport  Port=5  SampleTime=time_step
  wires:
  t_0/1 -> Normal obstacle ships trajectories prediction/6(t_0)
  Normal obstacle ships trajectories prediction/1(obstacle_ship_x_predicted) -> own_ship_obstacle_x_predicted/1, To Workspace4/1
  Normal obstacle ships trajectories prediction/2(obstacle_ship_y_predicted) -> own_ship_obstacle_y_predicted/1, To Workspace3/1
  own_ship_obstacle_headings/1 -> Normal obstacle ships trajectories prediction/1(obstacle_ship_psi)
  Normal obstacle ships trajectories prediction/5(obstacle_ship_psi_predicted) -> To Workspace2/1, own_ship_obstacle_psi_predicted/1
  Normal obstacle ships trajectories prediction/3(obstacle_ship_u_predicted) -> To Workspace1/1, own_ship_obstacle_u_predicted/1
  Normal obstacle ships trajectories prediction/4(obstacle_ship_v_predicted) -> To Workspace5/1, own_ship_obstacle_v_predicted/1
  own_ship_obstacle_u/1 -> Normal obstacle ships trajectories prediction/2(obstacle_ship_u)
  own_ship_obstacle_v/1 -> Normal obstacle ships trajectories prediction/3(obstacle_ship_v)
  own_ship_obstacle_x/1 -> Normal obstacle ships trajectories prediction/4(obstacle_ship_x)
  own_ship_obstacle_y/1 -> Normal obstacle ships trajectories prediction/5(obstacle_ship_y)

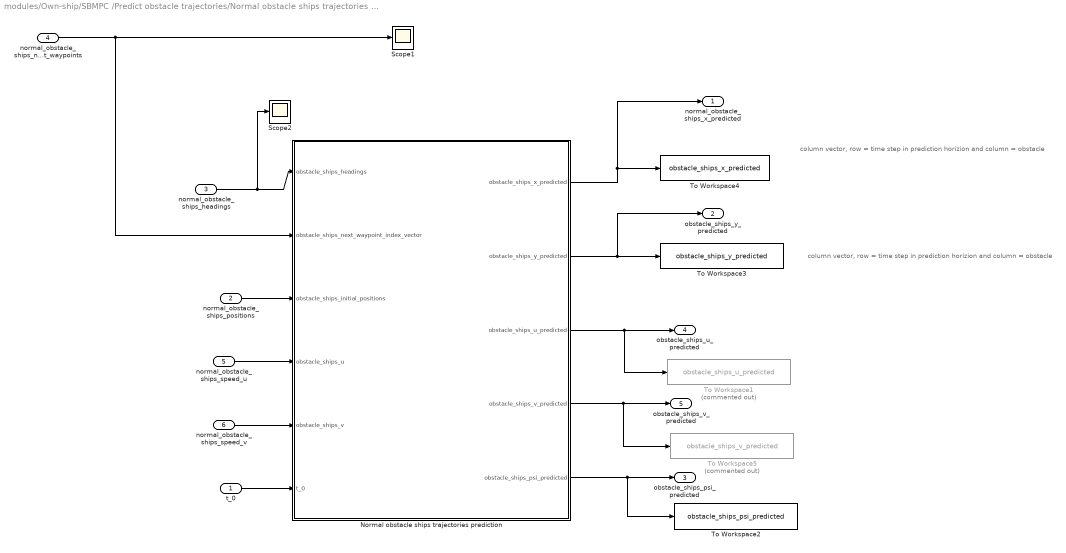
== system modules/Own-ship/SBMPC /Predict obstacle trajectories/Normal obstacle ships trajectories prediction ==
  note: column vector, row = time step in prediction horizion and column = obstacle
  note: column vector, row = time step in prediction horizion and column = obstacle
  t_0 : Inport
  normal_obstacle_ships_positions : Inport  Port=2
  normal_obstacle_ships_headings : Inport  Port=3
  normal_obstacle_ships_next_waypoints : Inport  Port=4
  normal_obstacle_ships_speed_u : Inport  Port=5
  normal_obstacle_ships_speed_v : Inport  Port=6
  Normal obstacle ships trajectories prediction : MATLAB Function  TreatAsAtomicUnit=on
  Scope1 : Scope
  Scope2 : Scope
  To Workspace1 : ToWorkspace  Commented=on  VariableName=obstacle_ships_u_predicted  SaveFormat=Structure With Time  SampleTime=tsamp
  To Workspace2 : ToWorkspace  VariableName=obstacle_ships_psi_predicted  SaveFormat=Structure With Time  SampleTime=tsamp
  To Workspace3 : ToWorkspace  VariableName=obstacle_ships_y_predicted  SaveFormat=Structure With Time  SampleTime=tsamp
  To Workspace4 : ToWorkspace  VariableName=obstacle_ships_x_predicted  SaveFormat=Structure With Time  SampleTime=tsamp
  To Workspace5 : ToWorkspace  Commented=on  VariableName=obstacle_ships_v_predicted  SaveFormat=Structure With Time  SampleTime=tsamp
  normal_obstacle_ships_x_predicted : Outport  SampleTime=time_step
  obstacle_ships_y_predicted : Outport  Port=2  SampleTime=time_step
  obstacle_ships_psi_predicted : Outport  Port=3  SampleTime=time_step
  obstacle_ships_u_predicted : Outport  Port=4  SampleTime=time_step
  obstacle_ships_v_predicted : Outport  Port=5  SampleTime=time_step
  wires:
  normal_obstacle_ships_positions/1 -> Normal obstacle ships trajectories prediction/3(obstacle_ships_initial_positions)
  normal_obstacle_ships_speed_v/1 -> Normal obstacle ships trajectories prediction/5(obstacle_ships_v)
  normal_obstacle_ships_speed_u/1 -> Normal obstacle ships trajectories prediction/4(obstacle_ships_u)
  t_0/1 -> Normal obstacle ships trajectories prediction/6(t_0)
  Normal obstacle ships trajectories prediction/1(obstacle_ships_x_predicted) -> normal_obstacle_ships_x_predicted/1, To Workspace4/1
  Normal obstacle ships trajectories prediction/2(obstacle_ships_y_predicted) -> obstacle_ships_y_predicted/1, To Workspace3/1
  normal_obstacle_ships_headings/1 -> Scope2/1, Normal obstacle ships trajectories prediction/1(obstacle_ships_headings)
  normal_obstacle_ships_next_waypoints/1 -> Normal obstacle ships trajectories prediction/2(obstacle_ships_next_waypoint_index_vector), Scope1/1
  Normal obstacle ships trajectories prediction/3(obstacle_ships_u_predicted) -> To Workspace1/1, obstacle_ships_u_predicted/1
  Normal obstacle ships trajectories prediction/5(obstacle_ships_psi_predicted) -> To Workspace2/1, obstacle_ships_psi_predicted/1
  Normal obstacle ships trajectories prediction/4(obstacle_ships_v_predicted) -> To Workspace5/1, obstacle_ships_v_predicted/1

== system modules/Own-ship/SBMPC /Predict obstacle trajectories/SBMPC obstacle ships trajectories prediction ==
  note: column vector, row = time step in prediction horizion and column = obstacle
  note: column vector, row = time step in prediction horizion and column = obstacle
  t_0 : Inport
  "SBMPC obstacle ships x " : Inport  Port=2
  "SBMPC obstacle ships y " : Inport  Port=3
  SBMPC obstacle ships psi : Inport  Port=4
  SBMPC obstacle ships u : Inport  Port=5
  SBMPC obstacle ships v : Inport  Port=6
  SBMPC obstacle ships trajectories prediction : MATLAB Function  TreatAsAtomicUnit=on
  To Workspace1 : ToWorkspace  Commented=on  VariableName=SBMPC_obstacle_ships_u_predicted  SaveFormat=Structure With Time  SampleTime=tsamp
  To Workspace2 : ToWorkspace  Commented=on  VariableName=SBMPC_obstacle_ships_psi_predicted  SaveFormat=Structure With Time  SampleTime=tsamp
  To Workspace3 : ToWorkspace  Commented=on  VariableName=SBMPC_obstacle_ships_y_predicted  SaveFormat=Structure With Time  SampleTime=tsamp
  To Workspace4 : ToWorkspace  Commented=on  VariableName=SBMPC_obstacle_ships_x_predicted  SaveFormat=Structure With Time  SampleTime=tsamp
  To Workspace5 : ToWorkspace  Commented=on  VariableName=SBMPC_obstacle_ships_v_predicted  SaveFormat=Structure With Time  SampleTime=tsamp
  SBMPC_obstacle_ships_x_predicted : Outport  SampleTime=time_step
  SBMPC_ships_y_predicted : Outport  Port=2  SampleTime=time_step
  SBMPC_ships_psi_predicted : Outport  Port=3  SampleTime=time_step
  SBMPC_ships_u_predicted : Outport  Port=4  SampleTime=time_step
  SBMPC_ships_v_predicted : Outport  Port=5  SampleTime=time_step
  wires:
  t_0/1 -> SBMPC obstacle ships trajectories prediction/6(t_0)
  SBMPC obstacle ships trajectories prediction/1(SBMPC_obstacle_ships_x_predicted) -> SBMPC_obstacle_ships_x_predicted/1, To Workspace4/1
  SBMPC obstacle ships trajectories prediction/2(SBMPC_obstacle_ships_y_predicted) -> SBMPC_ships_y_predicted/1, To Workspace3/1
  SBMPC obstacle ships trajectories prediction/3(SBMPC_obstacle_ships_u_predicted) -> To Workspace1/1, SBMPC_ships_u_predicted/1
  SBMPC obstacle ships trajectories prediction/5(SBMPC_obstacle_ships_psi_predicted) -> To Workspace2/1, SBMPC_ships_psi_predicted/1
  SBMPC obstacle ships trajectories prediction/4(SBMPC_obstacle_ships_v_predicted) -> To Workspace5/1, SBMPC_ships_v_predicted/1
  "SBMPC obstacle ships x "/1 -> SBMPC obstacle ships trajectories prediction/1(SBMPC_obstacle_ships_x)
  "SBMPC obstacle ships y "/1 -> SBMPC obstacle ships trajectories prediction/2(SBMPC_obstacle_ships_y)
  SBMPC obstacle ships psi/1 -> SBMPC obstacle ships trajectories prediction/3(SBMPC_obstacle_ships_psi)
  SBMPC obstacle ships u/1 -> SBMPC obstacle ships trajectories prediction/4(SBMPC_obstacle_ships_u)
  SBMPC obstacle ships v/1 -> SBMPC obstacle ships trajectories prediction/5(SBMPC_obstacle_ships_v)

== matlab function modules/Own-ship/vessel1/Vessel model/MATLAB Function ==
  data: Pr input; psi_ca input; desired_nu input; state output; desired_psi input; time_step parameter; eta_initial parameter; nu_initial parameter; tau output; Kp_feedback_linearization parameter; kp_heading parameter; Xmax parameter; Ymax parameter; Nmax parameter; K_sway parameter; K_yaw parameter; T_k_surge parameter; T_k_sway parameter; T_k_yaw parameter
function [state, tau]   = PSV(Pr, psi_ca, desired_nu, desired_psi, time_step, eta_initial, nu_initial, Kp_feedback_linearization, kp_heading, Xmax, Ymax, Nmax, K_sway, K_yaw, T_k_surge, T_k_sway, T_k_yaw)  
    desired_u = desired_nu(1);
    desired_v = desired_nu(2);
    desired_r = desired_nu(3);

    persistent psv_vessel; %Persistent variables are local to the function in which they are declared, yet their values are retained in memory between calls to the function.
    
    if (isempty(psv_vessel))
        psvParameters = coder.load('PSVparameters');
        psvModelParameters = psvParameters.model_config;
        psv_vessel = PSVvessel_class(psvModelParameters, eta_initial, nu_initial, time_step, desired_psi, desired_nu, Kp_feedback_linearization, kp_heading, Xmax, Ymax, Nmax, K_sway, K_yaw, T_k_surge, T_k_sway, T_k_yaw);
    end
    
    desired_psi = desired_psi + psi_ca;
    desired_nu(1) = desired_nu(1)*Pr;

    
    [psv_vessel, tau] = psv_vessel.update_states(desired_psi, desired_nu);           
    state = psv_vessel.state;   
end
